simulink model "demodOOK_done"  (R2018a)
settings: Solver=VariableStepAuto  StartTime=0.0  StopTime=10.0  RelTol=1e-3
model workspace (MAT data in the model file):
  MCOS : class17 (value not decoded)
  l = 39
  MCOS : class17 (value not decoded)
  rec : struct (value not decoded)
  tout = [0 2.08333333333e-05 4.16666666667e-05 6.25e-05 8.33333333333e-05 0.000104166666667 0.000125 0.000145833333333 0.000166666666667 0.0001875 0.000208333333333 0.000229166666667 ... (480001 elements, 480001x1)]
symbols that are objects in the model workspace (value not decoded): rec
libraries: simulink x3, commutil2 x2, simulink_need_slupdate x2, dspfdesign x2, dspsnks4 x1, rtlsdr_book_library x1, dspvision x1, dspstat3 x1, dspmtrx3 x1
(part 2 of 2)

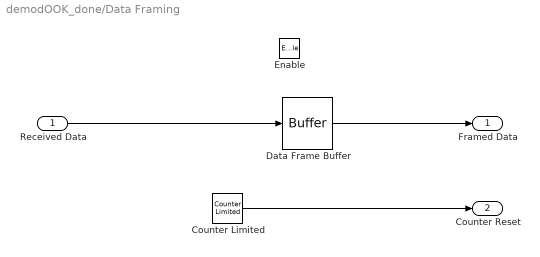
== system demodOOK_done/Data Framing ==
  Received Data : Inport
  Enable : EnablePort
  Counter Limited : simulink/Sources/Counter Limited  uplimit=rec.master_frame_len-rec.frame_pad_len-1  tsamp=-1
  Data Frame Buffer : Buffer  N=rec.master_frame_len-rec.frame_pad_len
  Framed Data : Outport
  Counter Reset : Outport  Port=2
  wires:
  Received Data/1 -> Data Frame Buffer/1
  Data Frame Buffer/1 -> Framed Data/1
  Counter Limited/1 -> Counter Reset/1

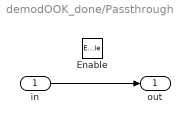
== system demodOOK_done/Passthrough ==
  in : Inport
  Enable : EnablePort
  out : Outport
  wires:
  in/1 -> out/1
